simulink model "TST_Rail_MonMeUn"  (R2016b)
settings: Solver=FixedStepDiscrete  StartTime=0.0  StopTime=simTime  FixedStep=sampleTime  RelTol=1e-3
values from neighbouring files (symbols this model uses):
  testCase = 1    [initTST_Rail_MonMeUn_001.m]    (also in initTST_Rail_MonMeUn_002.m = 2; initTST_Rail_MonMeUn_003.m = 3; initTST_Rail_MonMeUn_004.m = 4; initTST_Rail_MonMeUn_005.m = 5)
libraries: simulink x91, UnitTest_Lib x81
(part 3 of 5)

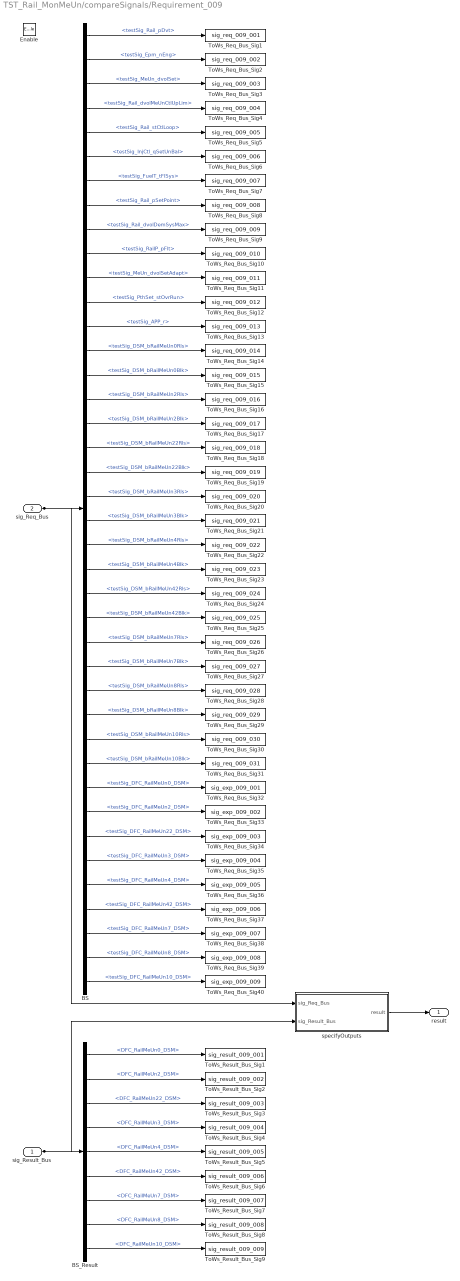
== system TST_Rail_MonMeUn/compareSignals/Requirement_009 ==
  sig_Result_Bus : Inport
  sig_Req_Bus : Inport  Port=2
  Enable : EnablePort
  BS : BusSelector  OutputSignals=testSig_Rail_pDvt,testSig_Epm_nEng,testSig_MeUn_dvolSet,testSig_Rail_dvolMeUnCtlUpLim,testSig_Rail_stCtlLoop,testSig_InjCtl_qSetUnBal,testSig_FuelT_tFlSys,testSig_Rail_pSetPoint,testSig_Rail_dvolDemSysMax,testSig_RailP_pFlt,testSig_MeUn_dvolSetAdapt,testSig_PthSet_stOvrRun,testSig_APP_r,testSig_DSM_bRailMeUn0Rls,testSig_DSM_bRailMeUn0Blk,testSig_DSM_bRailMeUn2Rls,testSig_DSM_bRailMeUn2Blk,testSig_DSM_bRailMeUn22Rls,testSig_DSM_bRailMeUn22Blk,testSig_DSM_bRailMeUn3Rls,testSig_DSM_bRailMeUn3Blk,testSig_DSM_bRailMeUn4Rls,testSig_DSM_bRailMeUn4Blk,testSig_DSM_bRailMeUn42Rls,testSig_DSM_bRailMeUn42Blk,testSig_DSM_bRailMeUn7Rls,testSig_DSM_bRailMeUn7Blk,testSig_DSM_bRailMeUn8Rls,testSig_DSM_bRailMeUn8Blk,testSig_DSM_bRailMeUn10Rls,testSig_DSM_bRailMeUn10Blk,testSig_DFC_RailMeUn0_DSM,testSig_DFC_RailMeUn2_DSM,testSig_DFC_RailMeUn22_DSM,testSig_DFC_RailMeUn3_DSM,testSig_DFC_RailMeUn4_DSM,testSig_DFC_RailMeUn42_DSM,testSig_DFC_RailMeUn7_DSM,testSig_DFC_RailMeUn8_DSM,testSig_DFC_RailMeUn10_DSM
  BS_Result : BusSelector  OutputSignals=DFC_RailMeUn0_DSM,DFC_RailMeUn2_DSM,DFC_RailMeUn22_DSM,DFC_RailMeUn3_DSM,DFC_RailMeUn4_DSM,DFC_RailMeUn42_DSM,DFC_RailMeUn7_DSM,DFC_RailMeUn8_DSM,DFC_RailMeUn10_DSM
  ToWs_Req_Bus_Sig1 : ToWorkspace  VariableName=sig_req_009_001  SaveFormat=Structure With Time
  ToWs_Req_Bus_Sig10 : ToWorkspace  VariableName=sig_req_009_010  SaveFormat=Structure With Time
  ToWs_Req_Bus_Sig11 : ToWorkspace  VariableName=sig_req_009_011  SaveFormat=Structure With Time
  ToWs_Req_Bus_Sig12 : ToWorkspace  VariableName=sig_req_009_012  SaveFormat=Structure With Time
  ToWs_Req_Bus_Sig13 : ToWorkspace  VariableName=sig_req_009_013  SaveFormat=Structure With Time
  ToWs_Req_Bus_Sig14 : ToWorkspace  VariableName=sig_req_009_014  SaveFormat=Structure With Time
  ToWs_Req_Bus_Sig15 : ToWorkspace  VariableName=sig_req_009_015  SaveFormat=Structure With Time
  ToWs_Req_Bus_Sig16 : ToWorkspace  VariableName=sig_req_009_016  SaveFormat=Structure With Time
  ToWs_Req_Bus_Sig17 : ToWorkspace  VariableName=sig_req_009_017  SaveFormat=Structure With Time
  ToWs_Req_Bus_Sig18 : ToWorkspace  VariableName=sig_req_009_018  SaveFormat=Structure With Time
  ToWs_Req_Bus_Sig19 : ToWorkspace  VariableName=sig_req_009_019  SaveFormat=Structure With Time
  ToWs_Req_Bus_Sig2 : ToWorkspace  VariableName=sig_req_009_002  SaveFormat=Structure With Time
  ToWs_Req_Bus_Sig20 : ToWorkspace  VariableName=sig_req_009_020  SaveFormat=Structure With Time
  ToWs_Req_Bus_Sig21 : ToWorkspace  VariableName=sig_req_009_021  SaveFormat=Structure With Time
  ToWs_Req_Bus_Sig22 : ToWorkspace  VariableName=sig_req_009_022  SaveFormat=Structure With Time
  ToWs_Req_Bus_Sig23 : ToWorkspace  VariableName=sig_req_009_023  SaveFormat=Structure With Time
  ToWs_Req_Bus_Sig24 : ToWorkspace  VariableName=sig_req_009_024  SaveFormat=Structure With Time
  ToWs_Req_Bus_Sig25 : ToWorkspace  VariableName=sig_req_009_025  SaveFormat=Structure With Time
  ToWs_Req_Bus_Sig26 : ToWorkspace  VariableName=sig_req_009_026  SaveFormat=Structure With Time
  ToWs_Req_Bus_Sig27 : ToWorkspace  VariableName=sig_req_009_027  SaveFormat=Structure With Time
  ToWs_Req_Bus_Sig28 : ToWorkspace  VariableName=sig_req_009_028  SaveFormat=Structure With Time
  ToWs_Req_Bus_Sig29 : ToWorkspace  VariableName=sig_req_009_029  SaveFormat=Structure With Time
  ToWs_Req_Bus_Sig3 : ToWorkspace  VariableName=sig_req_009_003  SaveFormat=Structure With Time
  ToWs_Req_Bus_Sig30 : ToWorkspace  VariableName=sig_req_009_030  SaveFormat=Structure With Time
  ToWs_Req_Bus_Sig31 : ToWorkspace  VariableName=sig_req_009_031  SaveFormat=Structure With Time
  ToWs_Req_Bus_Sig32 : ToWorkspace  VariableName=sig_exp_009_001  SaveFormat=Structure With Time
  ToWs_Req_Bus_Sig33 : ToWorkspace  VariableName=sig_exp_009_002  SaveFormat=Structure With Time
  ToWs_Req_Bus_Sig34 : ToWorkspace  VariableName=sig_exp_009_003  SaveFormat=Structure With Time
  ToWs_Req_Bus_Sig35 : ToWorkspace  VariableName=sig_exp_009_004  SaveFormat=Structure With Time
  ToWs_Req_Bus_Sig36 : ToWorkspace  VariableName=sig_exp_009_005  SaveFormat=Structure With Time
  ToWs_Req_Bus_Sig37 : ToWorkspace  VariableName=sig_exp_009_006  SaveFormat=Structure With Time
  ToWs_Req_Bus_Sig38 : ToWorkspace  VariableName=sig_exp_009_007  SaveFormat=Structure With Time
  ToWs_Req_Bus_Sig39 : ToWorkspace  VariableName=sig_exp_009_008  SaveFormat=Structure With Time
  ToWs_Req_Bus_Sig4 : ToWorkspace  VariableName=sig_req_009_004  SaveFormat=Structure With Time
  ToWs_Req_Bus_Sig40 : ToWorkspace  VariableName=sig_exp_009_009  SaveFormat=Structure With Time
  ToWs_Req_Bus_Sig5 : ToWorkspace  VariableName=sig_req_009_005  SaveFormat=Structure With Time
  ToWs_Req_Bus_Sig6 : ToWorkspace  VariableName=sig_req_009_006  SaveFormat=Structure With Time
  ToWs_Req_Bus_Sig7 : ToWorkspace  VariableName=sig_req_009_007  SaveFormat=Structure With Time
  ToWs_Req_Bus_Sig8 : ToWorkspace  VariableName=sig_req_009_008  SaveFormat=Structure With Time
  ToWs_Req_Bus_Sig9 : ToWorkspace  VariableName=sig_req_009_009  SaveFormat=Structure With Time
  ToWs_Result_Bus_Sig1 : ToWorkspace  VariableName=sig_result_009_001  SaveFormat=Structure With Time
  ToWs_Result_Bus_Sig2 : ToWorkspace  VariableName=sig_result_009_002  SaveFormat=Structure With Time
  ToWs_Result_Bus_Sig3 : ToWorkspace  VariableName=sig_result_009_003  SaveFormat=Structure With Time
  ToWs_Result_Bus_Sig4 : ToWorkspace  VariableName=sig_result_009_004  SaveFormat=Structure With Time
  ToWs_Result_Bus_Sig5 : ToWorkspace  VariableName=sig_result_009_005  SaveFormat=Structure With Time
  ToWs_Result_Bus_Sig6 : ToWorkspace  VariableName=sig_result_009_006  SaveFormat=Structure With Time
  ToWs_Result_Bus_Sig7 : ToWorkspace  VariableName=sig_result_009_007  SaveFormat=Structure With Time
  ToWs_Result_Bus_Sig8 : ToWorkspace  VariableName=sig_result_009_008  SaveFormat=Structure With Time
  ToWs_Result_Bus_Sig9 : ToWorkspace  VariableName=sig_result_009_009  SaveFormat=Structure With Time
  specifyOutputs : Subsystem
  result : Outport
  wires:
  sig_Req_Bus/1 -> BS/1, specifyOutputs/1(sig_Req_Bus)
  BS/1 -> ToWs_Req_Bus_Sig1/1  "<testSig_Rail_pDvt>"
  BS/2 -> ToWs_Req_Bus_Sig2/1  "<testSig_Epm_nEng>"
  BS/3 -> ToWs_Req_Bus_Sig3/1  "<testSig_MeUn_dvolSet>"
  BS/4 -> ToWs_Req_Bus_Sig4/1  "<testSig_Rail_dvolMeUnCtlUpLim>"
  BS/5 -> ToWs_Req_Bus_Sig5/1  "<testSig_Rail_stCtlLoop>"
  BS/6 -> ToWs_Req_Bus_Sig6/1  "<testSig_InjCtl_qSetUnBal>"
  BS/7 -> ToWs_Req_Bus_Sig7/1  "<testSig_FuelT_tFlSys>"
  BS/8 -> ToWs_Req_Bus_Sig8/1  "<testSig_Rail_pSetPoint>"
  BS/9 -> ToWs_Req_Bus_Sig9/1  "<testSig_Rail_dvolDemSysMax>"
  BS/10 -> ToWs_Req_Bus_Sig10/1  "<testSig_RailP_pFlt>"
  BS/11 -> ToWs_Req_Bus_Sig11/1  "<testSig_MeUn_dvolSetAdapt>"
  BS/12 -> ToWs_Req_Bus_Sig12/1  "<testSig_PthSet_stOvrRun>"
  BS/13 -> ToWs_Req_Bus_Sig13/1  "<testSig_APP_r>"
  BS/14 -> ToWs_Req_Bus_Sig14/1  "<testSig_DSM_bRailMeUn0Rls>"
  BS/15 -> ToWs_Req_Bus_Sig15/1  "<testSig_DSM_bRailMeUn0Blk>"
  BS/16 -> ToWs_Req_Bus_Sig16/1  "<testSig_DSM_bRailMeUn2Rls>"
  BS/17 -> ToWs_Req_Bus_Sig17/1  "<testSig_DSM_bRailMeUn2Blk>"
  BS/18 -> ToWs_Req_Bus_Sig18/1  "<testSig_DSM_bRailMeUn22Rls>"
  BS/19 -> ToWs_Req_Bus_Sig19/1  "<testSig_DSM_bRailMeUn22Blk>"
  BS/20 -> ToWs_Req_Bus_Sig20/1  "<testSig_DSM_bRailMeUn3Rls>"
  BS/21 -> ToWs_Req_Bus_Sig21/1  "<testSig_DSM_bRailMeUn3Blk>"
  BS/22 -> ToWs_Req_Bus_Sig22/1  "<testSig_DSM_bRailMeUn4Rls>"
  BS/23 -> ToWs_Req_Bus_Sig23/1  "<testSig_DSM_bRailMeUn4Blk>"
  BS/24 -> ToWs_Req_Bus_Sig24/1  "<testSig_DSM_bRailMeUn42Rls>"
  BS/25 -> ToWs_Req_Bus_Sig25/1  "<testSig_DSM_bRailMeUn42Blk>"
  BS/26 -> ToWs_Req_Bus_Sig26/1  "<testSig_DSM_bRailMeUn7Rls>"
  BS/27 -> ToWs_Req_Bus_Sig27/1  "<testSig_DSM_bRailMeUn7Blk>"
  BS/28 -> ToWs_Req_Bus_Sig28/1  "<testSig_DSM_bRailMeUn8Rls>"
  BS/29 -> ToWs_Req_Bus_Sig29/1  "<testSig_DSM_bRailMeUn8Blk>"
  BS/30 -> ToWs_Req_Bus_Sig30/1  "<testSig_DSM_bRailMeUn10Rls>"
  BS/31 -> ToWs_Req_Bus_Sig31/1  "<testSig_DSM_bRailMeUn10Blk>"
  BS/32 -> ToWs_Req_Bus_Sig32/1  "<testSig_DFC_RailMeUn0_DSM>"
  BS/33 -> ToWs_Req_Bus_Sig33/1  "<testSig_DFC_RailMeUn2_DSM>"
  BS/34 -> ToWs_Req_Bus_Sig34/1  "<testSig_DFC_RailMeUn22_DSM>"
  BS/35 -> ToWs_Req_Bus_Sig35/1  "<testSig_DFC_RailMeUn3_DSM>"
  BS/36 -> ToWs_Req_Bus_Sig36/1  "<testSig_DFC_RailMeUn4_DSM>"
  BS/37 -> ToWs_Req_Bus_Sig37/1  "<testSig_DFC_RailMeUn42_DSM>"
  BS/38 -> ToWs_Req_Bus_Sig38/1  "<testSig_DFC_RailMeUn7_DSM>"
  BS/39 -> ToWs_Req_Bus_Sig39/1  "<testSig_DFC_RailMeUn8_DSM>"
  BS/40 -> ToWs_Req_Bus_Sig40/1  "<testSig_DFC_RailMeUn10_DSM>"
  sig_Result_Bus/1 -> BS_Result/1, specifyOutputs/2(sig_Result_Bus)
  BS_Result/1 -> ToWs_Result_Bus_Sig1/1  "<DFC_RailMeUn0_DSM>"
  BS_Result/2 -> ToWs_Result_Bus_Sig2/1  "<DFC_RailMeUn2_DSM>"
  BS_Result/3 -> ToWs_Result_Bus_Sig3/1  "<DFC_RailMeUn22_DSM>"
  BS_Result/4 -> ToWs_Result_Bus_Sig4/1  "<DFC_RailMeUn3_DSM>"
  BS_Result/5 -> ToWs_Result_Bus_Sig5/1  "<DFC_RailMeUn4_DSM>"
  BS_Result/6 -> ToWs_Result_Bus_Sig6/1  "<DFC_RailMeUn42_DSM>"
  BS_Result/7 -> ToWs_Result_Bus_Sig7/1  "<DFC_RailMeUn7_DSM>"
  BS_Result/8 -> ToWs_Result_Bus_Sig8/1  "<DFC_RailMeUn8_DSM>"
  BS_Result/9 -> ToWs_Result_Bus_Sig9/1  "<DFC_RailMeUn10_DSM>"
  specifyOutputs/1(result) -> result/1

== system TST_Rail_MonMeUn/simulationInput/testSignals_R001 ==
  BC : BusCreator  Inputs=40
  spec_APP_r : FromWorkspace  VariableName=testSig_APP_r  Interpolate=off  OutputAfterFinalValue=Holding final value
  spec_DFC_RailMeUn0_DSM : FromWorkspace  VariableName=testSig_DFC_RailMeUn0_DSM  Interpolate=off  OutputAfterFinalValue=Holding final value
  spec_DFC_RailMeUn10_DSM : FromWorkspace  VariableName=testSig_DFC_RailMeUn10_DSM  Interpolate=off  OutputAfterFinalValue=Holding final value
  spec_DFC_RailMeUn22_DSM : FromWorkspace  VariableName=testSig_DFC_RailMeUn22_DSM  Interpolate=off  OutputAfterFinalValue=Holding final value
  spec_DFC_RailMeUn2_DSM : FromWorkspace  VariableName=testSig_DFC_RailMeUn2_DSM  Interpolate=off  OutputAfterFinalValue=Holding final value
  spec_DFC_RailMeUn3_DSM : FromWorkspace  VariableName=testSig_DFC_RailMeUn3_DSM  Interpolate=off  OutputAfterFinalValue=Holding final value
  spec_DFC_RailMeUn42_DSM : FromWorkspace  VariableName=testSig_DFC_RailMeUn42_DSM  Interpolate=off  OutputAfterFinalValue=Holding final value
  spec_DFC_RailMeUn4_DSM : FromWorkspace  VariableName=testSig_DFC_RailMeUn4_DSM  Interpolate=off  OutputAfterFinalValue=Holding final value
  spec_DFC_RailMeUn7_DSM : FromWorkspace  VariableName=testSig_DFC_RailMeUn7_DSM  Interpolate=off  OutputAfterFinalValue=Holding final value
  spec_DFC_RailMeUn8_DSM : FromWorkspace  VariableName=testSig_DFC_RailMeUn8_DSM  Interpolate=off  OutputAfterFinalValue=Holding final value
  spec_DSM_bRailMeUn0Blk : FromWorkspace  VariableName=testSig_DSM_bRailMeUn0Blk  Interpolate=off  OutputAfterFinalValue=Holding final value
  spec_DSM_bRailMeUn0Rls : FromWorkspace  VariableName=testSig_DSM_bRailMeUn0Rls  Interpolate=off  OutputAfterFinalValue=Holding final value
  spec_DSM_bRailMeUn10Blk : FromWorkspace  VariableName=testSig_DSM_bRailMeUn10Blk  Interpolate=off  OutputAfterFinalValue=Holding final value
  spec_DSM_bRailMeUn10Rls : FromWorkspace  VariableName=testSig_DSM_bRailMeUn10Rls  Interpolate=off  OutputAfterFinalValue=Holding final value
  spec_DSM_bRailMeUn22Blk : FromWorkspace  VariableName=testSig_DSM_bRailMeUn22Blk  Interpolate=off  OutputAfterFinalValue=Holding final value
  spec_DSM_bRailMeUn22Rls : FromWorkspace  VariableName=testSig_DSM_bRailMeUn22Rls  Interpolate=off  OutputAfterFinalValue=Holding final value
  spec_DSM_bRailMeUn2Blk : FromWorkspace  VariableName=testSig_DSM_bRailMeUn2Blk  Interpolate=off  OutputAfterFinalValue=Holding final value
  spec_DSM_bRailMeUn2Rls : FromWorkspace  VariableName=testSig_DSM_bRailMeUn2Rls  Interpolate=off  OutputAfterFinalValue=Holding final value
  spec_DSM_bRailMeUn3Blk : FromWorkspace  VariableName=testSig_DSM_bRailMeUn3Blk  Interpolate=off  OutputAfterFinalValue=Holding final value
  spec_DSM_bRailMeUn3Rls : FromWorkspace  VariableName=testSig_DSM_bRailMeUn3Rls  Interpolate=off  OutputAfterFinalValue=Holding final value
  spec_DSM_bRailMeUn42Blk : FromWorkspace  VariableName=testSig_DSM_bRailMeUn42Blk  Interpolate=off  OutputAfterFinalValue=Holding final value
  spec_DSM_bRailMeUn42Rls : FromWorkspace  VariableName=testSig_DSM_bRailMeUn42Rls  Interpolate=off  OutputAfterFinalValue=Holding final value
  spec_DSM_bRailMeUn4Blk : FromWorkspace  VariableName=testSig_DSM_bRailMeUn4Blk  Interpolate=off  OutputAfterFinalValue=Holding final value
  spec_DSM_bRailMeUn4Rls : FromWorkspace  VariableName=testSig_DSM_bRailMeUn4Rls  Interpolate=off  OutputAfterFinalValue=Holding final value
  spec_DSM_bRailMeUn7Blk : FromWorkspace  VariableName=testSig_DSM_bRailMeUn7Blk  Interpolate=off  OutputAfterFinalValue=Holding final value
  spec_DSM_bRailMeUn7Rls : FromWorkspace  VariableName=testSig_DSM_bRailMeUn7Rls  Interpolate=off  OutputAfterFinalValue=Holding final value
  spec_DSM_bRailMeUn8Blk : FromWorkspace  VariableName=testSig_DSM_bRailMeUn8Blk  Interpolate=off  OutputAfterFinalValue=Holding final value
  spec_DSM_bRailMeUn8Rls : FromWorkspace  VariableName=testSig_DSM_bRailMeUn8Rls  Interpolate=off  OutputAfterFinalValue=Holding final value
  spec_Epm_nEng : FromWorkspace  VariableName=testSig_Epm_nEng  Interpolate=off  OutputAfterFinalValue=Holding final value
  spec_FuelT_tFlSys : FromWorkspace  VariableName=testSig_FuelT_tFlSys  Interpolate=off  OutputAfterFinalValue=Holding final value
  spec_InjCtl_qSetUnBal : FromWorkspace  VariableName=testSig_InjCtl_qSetUnBal  Interpolate=off  OutputAfterFinalValue=Holding final value
  spec_MeUn_dvolSet : FromWorkspace  VariableName=testSig_MeUn_dvolSet  Interpolate=off  OutputAfterFinalValue=Holding final value
  spec_MeUn_dvolSetAdapt : FromWorkspace  VariableName=testSig_MeUn_dvolSetAdapt  Interpolate=off  OutputAfterFinalValue=Holding final value
  spec_PthSet_stOvrRun : FromWorkspace  VariableName=testSig_PthSet_stOvrRun  Interpolate=off  OutputAfterFinalValue=Holding final value
  spec_RailP_pFlt : FromWorkspace  VariableName=testSig_RailP_pFlt  Interpolate=off  OutputAfterFinalValue=Holding final value
  spec_Rail_dvolDemSysMax : FromWorkspace  VariableName=testSig_Rail_dvolDemSysMax  Interpolate=off  OutputAfterFinalValue=Holding final value
  spec_Rail_dvolMeUnCtlUpLim : FromWorkspace  VariableName=testSig_Rail_dvolMeUnCtlUpLim  Interpolate=off  OutputAfterFinalValue=Holding final value
  spec_Rail_pDvt : FromWorkspace  VariableName=testSig_Rail_pDvt  Interpolate=off  OutputAfterFinalValue=Holding final value
  spec_Rail_pSetPoint : FromWorkspace  VariableName=testSig_Rail_pSetPoint  Interpolate=off  OutputAfterFinalValue=Holding final value
  spec_Rail_stCtlLoop : FromWorkspace  VariableName=testSig_Rail_stCtlLoop  Interpolate=off  OutputAfterFinalValue=Holding final value
  testSignals : Outport
  wires:
  BC/1 -> testSignals/1
  spec_Rail_pDvt/1 -> BC/1  "testSig_Rail_pDvt"
  spec_Epm_nEng/1 -> BC/2  "testSig_Epm_nEng"
  spec_MeUn_dvolSet/1 -> BC/3  "testSig_MeUn_dvolSet"
  spec_Rail_dvolMeUnCtlUpLim/1 -> BC/4  "testSig_Rail_dvolMeUnCtlUpLim"
  spec_Rail_stCtlLoop/1 -> BC/5  "testSig_Rail_stCtlLoop"
  spec_InjCtl_qSetUnBal/1 -> BC/6  "testSig_InjCtl_qSetUnBal"
  spec_FuelT_tFlSys/1 -> BC/7  "testSig_FuelT_tFlSys"
  spec_Rail_pSetPoint/1 -> BC/8  "testSig_Rail_pSetPoint"
  spec_Rail_dvolDemSysMax/1 -> BC/9  "testSig_Rail_dvolDemSysMax"
  spec_RailP_pFlt/1 -> BC/10  "testSig_RailP_pFlt"
  spec_MeUn_dvolSetAdapt/1 -> BC/11  "testSig_MeUn_dvolSetAdapt"
  spec_PthSet_stOvrRun/1 -> BC/12  "testSig_PthSet_stOvrRun"
  spec_APP_r/1 -> BC/13  "testSig_APP_r"
  spec_DSM_bRailMeUn0Rls/1 -> BC/14  "testSig_DSM_bRailMeUn0Rls"
  spec_DSM_bRailMeUn0Blk/1 -> BC/15  "testSig_DSM_bRailMeUn0Blk"
  spec_DSM_bRailMeUn2Rls/1 -> BC/16  "testSig_DSM_bRailMeUn2Rls"
  spec_DSM_bRailMeUn2Blk/1 -> BC/17  "testSig_DSM_bRailMeUn2Blk"
  spec_DSM_bRailMeUn22Rls/1 -> BC/18  "testSig_DSM_bRailMeUn22Rls"
  spec_DSM_bRailMeUn22Blk/1 -> BC/19  "testSig_DSM_bRailMeUn22Blk"
  spec_DSM_bRailMeUn3Rls/1 -> BC/20  "testSig_DSM_bRailMeUn3Rls"
  spec_DSM_bRailMeUn3Blk/1 -> BC/21  "testSig_DSM_bRailMeUn3Blk"
  spec_DSM_bRailMeUn4Rls/1 -> BC/22  "testSig_DSM_bRailMeUn4Rls"
  spec_DSM_bRailMeUn4Blk/1 -> BC/23  "testSig_DSM_bRailMeUn4Blk"
  spec_DSM_bRailMeUn42Rls/1 -> BC/24  "testSig_DSM_bRailMeUn42Rls"
  spec_DSM_bRailMeUn42Blk/1 -> BC/25  "testSig_DSM_bRailMeUn42Blk"
  spec_DSM_bRailMeUn7Rls/1 -> BC/26  "testSig_DSM_bRailMeUn7Rls"
  spec_DSM_bRailMeUn7Blk/1 -> BC/27  "testSig_DSM_bRailMeUn7Blk"
  spec_DSM_bRailMeUn8Rls/1 -> BC/28  "testSig_DSM_bRailMeUn8Rls"
  spec_DSM_bRailMeUn8Blk/1 -> BC/29  "testSig_DSM_bRailMeUn8Blk"
  spec_DSM_bRailMeUn10Rls/1 -> BC/30  "testSig_DSM_bRailMeUn10Rls"
  spec_DSM_bRailMeUn10Blk/1 -> BC/31  "testSig_DSM_bRailMeUn10Blk"
  spec_DFC_RailMeUn0_DSM/1 -> BC/32  "testSig_DFC_RailMeUn0_DSM"
  spec_DFC_RailMeUn2_DSM/1 -> BC/33  "testSig_DFC_RailMeUn2_DSM"
  spec_DFC_RailMeUn22_DSM/1 -> BC/34  "testSig_DFC_RailMeUn22_DSM"
  spec_DFC_RailMeUn3_DSM/1 -> BC/35  "testSig_DFC_RailMeUn3_DSM"
  spec_DFC_RailMeUn4_DSM/1 -> BC/36  "testSig_DFC_RailMeUn4_DSM"
  spec_DFC_RailMeUn42_DSM/1 -> BC/37  "testSig_DFC_RailMeUn42_DSM"
  spec_DFC_RailMeUn7_DSM/1 -> BC/38  "testSig_DFC_RailMeUn7_DSM"
  spec_DFC_RailMeUn8_DSM/1 -> BC/39  "testSig_DFC_RailMeUn8_DSM"
  spec_DFC_RailMeUn10_DSM/1 -> BC/40  "testSig_DFC_RailMeUn10_DSM"

== system TST_Rail_MonMeUn/simulationInput/testSignals_R002 ==
  BC : BusCreator  Inputs=40
  spec_APP_r : FromWorkspace  VariableName=testSig_APP_r  Interpolate=off  OutputAfterFinalValue=Holding final value
  spec_DFC_RailMeUn0_DSM : FromWorkspace  VariableName=testSig_DFC_RailMeUn0_DSM  Interpolate=off  OutputAfterFinalValue=Holding final value
  spec_DFC_RailMeUn10_DSM : FromWorkspace  VariableName=testSig_DFC_RailMeUn10_DSM  Interpolate=off  OutputAfterFinalValue=Holding final value
  spec_DFC_RailMeUn22_DSM : FromWorkspace  VariableName=testSig_DFC_RailMeUn22_DSM  Interpolate=off  OutputAfterFinalValue=Holding final value
  spec_DFC_RailMeUn2_DSM : FromWorkspace  VariableName=testSig_DFC_RailMeUn2_DSM  Interpolate=off  OutputAfterFinalValue=Holding final value
  spec_DFC_RailMeUn3_DSM : FromWorkspace  VariableName=testSig_DFC_RailMeUn3_DSM  Interpolate=off  OutputAfterFinalValue=Holding final value
  spec_DFC_RailMeUn42_DSM : FromWorkspace  VariableName=testSig_DFC_RailMeUn42_DSM  Interpolate=off  OutputAfterFinalValue=Holding final value
  spec_DFC_RailMeUn4_DSM : FromWorkspace  VariableName=testSig_DFC_RailMeUn4_DSM  Interpolate=off  OutputAfterFinalValue=Holding final value
  spec_DFC_RailMeUn7_DSM : FromWorkspace  VariableName=testSig_DFC_RailMeUn7_DSM  Interpolate=off  OutputAfterFinalValue=Holding final value
  spec_DFC_RailMeUn8_DSM : FromWorkspace  VariableName=testSig_DFC_RailMeUn8_DSM  Interpolate=off  OutputAfterFinalValue=Holding final value
  spec_DSM_bRailMeUn0Blk : FromWorkspace  VariableName=testSig_DSM_bRailMeUn0Blk  Interpolate=off  OutputAfterFinalValue=Holding final value
  spec_DSM_bRailMeUn0Rls : FromWorkspace  VariableName=testSig_DSM_bRailMeUn0Rls  Interpolate=off  OutputAfterFinalValue=Holding final value
  spec_DSM_bRailMeUn10Blk : FromWorkspace  VariableName=testSig_DSM_bRailMeUn10Blk  Interpolate=off  OutputAfterFinalValue=Holding final value
  spec_DSM_bRailMeUn10Rls : FromWorkspace  VariableName=testSig_DSM_bRailMeUn10Rls  Interpolate=off  OutputAfterFinalValue=Holding final value
  spec_DSM_bRailMeUn22Blk : FromWorkspace  VariableName=testSig_DSM_bRailMeUn22Blk  Interpolate=off  OutputAfterFinalValue=Holding final value
  spec_DSM_bRailMeUn22Rls : FromWorkspace  VariableName=testSig_DSM_bRailMeUn22Rls  Interpolate=off  OutputAfterFinalValue=Holding final value
  spec_DSM_bRailMeUn2Blk : FromWorkspace  VariableName=testSig_DSM_bRailMeUn2Blk  Interpolate=off  OutputAfterFinalValue=Holding final value
  spec_DSM_bRailMeUn2Rls : FromWorkspace  VariableName=testSig_DSM_bRailMeUn2Rls  Interpolate=off  OutputAfterFinalValue=Holding final value
  spec_DSM_bRailMeUn3Blk : FromWorkspace  VariableName=testSig_DSM_bRailMeUn3Blk  Interpolate=off  OutputAfterFinalValue=Holding final value
  spec_DSM_bRailMeUn3Rls : FromWorkspace  VariableName=testSig_DSM_bRailMeUn3Rls  Interpolate=off  OutputAfterFinalValue=Holding final value
  spec_DSM_bRailMeUn42Blk : FromWorkspace  VariableName=testSig_DSM_bRailMeUn42Blk  Interpolate=off  OutputAfterFinalValue=Holding final value
  spec_DSM_bRailMeUn42Rls : FromWorkspace  VariableName=testSig_DSM_bRailMeUn42Rls  Interpolate=off  OutputAfterFinalValue=Holding final value
  spec_DSM_bRailMeUn4Blk : FromWorkspace  VariableName=testSig_DSM_bRailMeUn4Blk  Interpolate=off  OutputAfterFinalValue=Holding final value
  spec_DSM_bRailMeUn4Rls : FromWorkspace  VariableName=testSig_DSM_bRailMeUn4Rls  Interpolate=off  OutputAfterFinalValue=Holding final value
  spec_DSM_bRailMeUn7Blk : FromWorkspace  VariableName=testSig_DSM_bRailMeUn7Blk  Interpolate=off  OutputAfterFinalValue=Holding final value
  spec_DSM_bRailMeUn7Rls : FromWorkspace  VariableName=testSig_DSM_bRailMeUn7Rls  Interpolate=off  OutputAfterFinalValue=Holding final value
  spec_DSM_bRailMeUn8Blk : FromWorkspace  VariableName=testSig_DSM_bRailMeUn8Blk  Interpolate=off  OutputAfterFinalValue=Holding final value
  spec_DSM_bRailMeUn8Rls : FromWorkspace  VariableName=testSig_DSM_bRailMeUn8Rls  Interpolate=off  OutputAfterFinalValue=Holding final value
  spec_Epm_nEng : FromWorkspace  VariableName=testSig_Epm_nEng  Interpolate=off  OutputAfterFinalValue=Holding final value
  spec_FuelT_tFlSys : FromWorkspace  VariableName=testSig_FuelT_tFlSys  Interpolate=off  OutputAfterFinalValue=Holding final value
  spec_InjCtl_qSetUnBal : FromWorkspace  VariableName=testSig_InjCtl_qSetUnBal  Interpolate=off  OutputAfterFinalValue=Holding final value
  spec_MeUn_dvolSet : FromWorkspace  VariableName=testSig_MeUn_dvolSet  Interpolate=off  OutputAfterFinalValue=Holding final value
  spec_MeUn_dvolSetAdapt : FromWorkspace  VariableName=testSig_MeUn_dvolSetAdapt  Interpolate=off  OutputAfterFinalValue=Holding final value
  spec_PthSet_stOvrRun : FromWorkspace  VariableName=testSig_PthSet_stOvrRun  Interpolate=off  OutputAfterFinalValue=Holding final value
  spec_RailP_pFlt : FromWorkspace  VariableName=testSig_RailP_pFlt  Interpolate=off  OutputAfterFinalValue=Holding final value
  spec_Rail_dvolDemSysMax : FromWorkspace  VariableName=testSig_Rail_dvolDemSysMax  Interpolate=off  OutputAfterFinalValue=Holding final value
  spec_Rail_dvolMeUnCtlUpLim : FromWorkspace  VariableName=testSig_Rail_dvolMeUnCtlUpLim  Interpolate=off  OutputAfterFinalValue=Holding final value
  spec_Rail_pDvt : FromWorkspace  VariableName=testSig_Rail_pDvt  Interpolate=off  OutputAfterFinalValue=Holding final value
  spec_Rail_pSetPoint : FromWorkspace  VariableName=testSig_Rail_pSetPoint  Interpolate=off  OutputAfterFinalValue=Holding final value
  spec_Rail_stCtlLoop : FromWorkspace  VariableName=testSig_Rail_stCtlLoop  Interpolate=off  OutputAfterFinalValue=Holding final value
  testSignals : Outport
  wires:
  BC/1 -> testSignals/1
  spec_Rail_pDvt/1 -> BC/1  "testSig_Rail_pDvt"
  spec_Epm_nEng/1 -> BC/2  "testSig_Epm_nEng"
  spec_MeUn_dvolSet/1 -> BC/3  "testSig_MeUn_dvolSet"
  spec_Rail_dvolMeUnCtlUpLim/1 -> BC/4  "testSig_Rail_dvolMeUnCtlUpLim"
  spec_Rail_stCtlLoop/1 -> BC/5  "testSig_Rail_stCtlLoop"
  spec_InjCtl_qSetUnBal/1 -> BC/6  "testSig_InjCtl_qSetUnBal"
  spec_FuelT_tFlSys/1 -> BC/7  "testSig_FuelT_tFlSys"
  spec_Rail_pSetPoint/1 -> BC/8  "testSig_Rail_pSetPoint"
  spec_Rail_dvolDemSysMax/1 -> BC/9  "testSig_Rail_dvolDemSysMax"
  spec_RailP_pFlt/1 -> BC/10  "testSig_RailP_pFlt"
  spec_MeUn_dvolSetAdapt/1 -> BC/11  "testSig_MeUn_dvolSetAdapt"
  spec_PthSet_stOvrRun/1 -> BC/12  "testSig_PthSet_stOvrRun"
  spec_APP_r/1 -> BC/13  "testSig_APP_r"
  spec_DSM_bRailMeUn0Rls/1 -> BC/14  "testSig_DSM_bRailMeUn0Rls"
  spec_DSM_bRailMeUn0Blk/1 -> BC/15  "testSig_DSM_bRailMeUn0Blk"
  spec_DSM_bRailMeUn2Rls/1 -> BC/16  "testSig_DSM_bRailMeUn2Rls"
  spec_DSM_bRailMeUn2Blk/1 -> BC/17  "testSig_DSM_bRailMeUn2Blk"
  spec_DSM_bRailMeUn22Rls/1 -> BC/18  "testSig_DSM_bRailMeUn22Rls"
  spec_DSM_bRailMeUn22Blk/1 -> BC/19  "testSig_DSM_bRailMeUn22Blk"
  spec_DSM_bRailMeUn3Rls/1 -> BC/20  "testSig_DSM_bRailMeUn3Rls"
  spec_DSM_bRailMeUn3Blk/1 -> BC/21  "testSig_DSM_bRailMeUn3Blk"
  spec_DSM_bRailMeUn4Rls/1 -> BC/22  "testSig_DSM_bRailMeUn4Rls"
  spec_DSM_bRailMeUn4Blk/1 -> BC/23  "testSig_DSM_bRailMeUn4Blk"
  spec_DSM_bRailMeUn42Rls/1 -> BC/24  "testSig_DSM_bRailMeUn42Rls"
  spec_DSM_bRailMeUn42Blk/1 -> BC/25  "testSig_DSM_bRailMeUn42Blk"
  spec_DSM_bRailMeUn7Rls/1 -> BC/26  "testSig_DSM_bRailMeUn7Rls"
  spec_DSM_bRailMeUn7Blk/1 -> BC/27  "testSig_DSM_bRailMeUn7Blk"
  spec_DSM_bRailMeUn8Rls/1 -> BC/28  "testSig_DSM_bRailMeUn8Rls"
  spec_DSM_bRailMeUn8Blk/1 -> BC/29  "testSig_DSM_bRailMeUn8Blk"
  spec_DSM_bRailMeUn10Rls/1 -> BC/30  "testSig_DSM_bRailMeUn10Rls"
  spec_DSM_bRailMeUn10Blk/1 -> BC/31  "testSig_DSM_bRailMeUn10Blk"
  spec_DFC_RailMeUn0_DSM/1 -> BC/32  "testSig_DFC_RailMeUn0_DSM"
  spec_DFC_RailMeUn2_DSM/1 -> BC/33  "testSig_DFC_RailMeUn2_DSM"
  spec_DFC_RailMeUn22_DSM/1 -> BC/34  "testSig_DFC_RailMeUn22_DSM"
  spec_DFC_RailMeUn3_DSM/1 -> BC/35  "testSig_DFC_RailMeUn3_DSM"
  spec_DFC_RailMeUn4_DSM/1 -> BC/36  "testSig_DFC_RailMeUn4_DSM"
  spec_DFC_RailMeUn42_DSM/1 -> BC/37  "testSig_DFC_RailMeUn42_DSM"
  spec_DFC_RailMeUn7_DSM/1 -> BC/38  "testSig_DFC_RailMeUn7_DSM"
  spec_DFC_RailMeUn8_DSM/1 -> BC/39  "testSig_DFC_RailMeUn8_DSM"
  spec_DFC_RailMeUn10_DSM/1 -> BC/40  "testSig_DFC_RailMeUn10_DSM"

== system TST_Rail_MonMeUn/simulationInput/testSignals_R003 ==
  BC : BusCreator  Inputs=40
  spec_APP_r : FromWorkspace  VariableName=testSig_APP_r  Interpolate=off  OutputAfterFinalValue=Holding final value
  spec_DFC_RailMeUn0_DSM : FromWorkspace  VariableName=testSig_DFC_RailMeUn0_DSM  Interpolate=off  OutputAfterFinalValue=Holding final value
  spec_DFC_RailMeUn10_DSM : FromWorkspace  VariableName=testSig_DFC_RailMeUn10_DSM  Interpolate=off  OutputAfterFinalValue=Holding final value
  spec_DFC_RailMeUn22_DSM : FromWorkspace  VariableName=testSig_DFC_RailMeUn22_DSM  Interpolate=off  OutputAfterFinalValue=Holding final value
  spec_DFC_RailMeUn2_DSM : FromWorkspace  VariableName=testSig_DFC_RailMeUn2_DSM  Interpolate=off  OutputAfterFinalValue=Holding final value
  spec_DFC_RailMeUn3_DSM : FromWorkspace  VariableName=testSig_DFC_RailMeUn3_DSM  Interpolate=off  OutputAfterFinalValue=Holding final value
  spec_DFC_RailMeUn42_DSM : FromWorkspace  VariableName=testSig_DFC_RailMeUn42_DSM  Interpolate=off  OutputAfterFinalValue=Holding final value
  spec_DFC_RailMeUn4_DSM : FromWorkspace  VariableName=testSig_DFC_RailMeUn4_DSM  Interpolate=off  OutputAfterFinalValue=Holding final value
  spec_DFC_RailMeUn7_DSM : FromWorkspace  VariableName=testSig_DFC_RailMeUn7_DSM  Interpolate=off  OutputAfterFinalValue=Holding final value
  spec_DFC_RailMeUn8_DSM : FromWorkspace  VariableName=testSig_DFC_RailMeUn8_DSM  Interpolate=off  OutputAfterFinalValue=Holding final value
  spec_DSM_bRailMeUn0Blk : FromWorkspace  VariableName=testSig_DSM_bRailMeUn0Blk  Interpolate=off  OutputAfterFinalValue=Holding final value
  spec_DSM_bRailMeUn0Rls : FromWorkspace  VariableName=testSig_DSM_bRailMeUn0Rls  Interpolate=off  OutputAfterFinalValue=Holding final value
  spec_DSM_bRailMeUn10Blk : FromWorkspace  VariableName=testSig_DSM_bRailMeUn10Blk  Interpolate=off  OutputAfterFinalValue=Holding final value
  spec_DSM_bRailMeUn10Rls : FromWorkspace  VariableName=testSig_DSM_bRailMeUn10Rls  Interpolate=off  OutputAfterFinalValue=Holding final value
  spec_DSM_bRailMeUn22Blk : FromWorkspace  VariableName=testSig_DSM_bRailMeUn22Blk  Interpolate=off  OutputAfterFinalValue=Holding final value
  spec_DSM_bRailMeUn22Rls : FromWorkspace  VariableName=testSig_DSM_bRailMeUn22Rls  Interpolate=off  OutputAfterFinalValue=Holding final value
  spec_DSM_bRailMeUn2Blk : FromWorkspace  VariableName=testSig_DSM_bRailMeUn2Blk  Interpolate=off  OutputAfterFinalValue=Holding final value
  spec_DSM_bRailMeUn2Rls : FromWorkspace  VariableName=testSig_DSM_bRailMeUn2Rls  Interpolate=off  OutputAfterFinalValue=Holding final value
  spec_DSM_bRailMeUn3Blk : FromWorkspace  VariableName=testSig_DSM_bRailMeUn3Blk  Interpolate=off  OutputAfterFinalValue=Holding final value
  spec_DSM_bRailMeUn3Rls : FromWorkspace  VariableName=testSig_DSM_bRailMeUn3Rls  Interpolate=off  OutputAfterFinalValue=Holding final value
  spec_DSM_bRailMeUn42Blk : FromWorkspace  VariableName=testSig_DSM_bRailMeUn42Blk  Interpolate=off  OutputAfterFinalValue=Holding final value
  spec_DSM_bRailMeUn42Rls : FromWorkspace  VariableName=testSig_DSM_bRailMeUn42Rls  Interpolate=off  OutputAfterFinalValue=Holding final value
  spec_DSM_bRailMeUn4Blk : FromWorkspace  VariableName=testSig_DSM_bRailMeUn4Blk  Interpolate=off  OutputAfterFinalValue=Holding final value
  spec_DSM_bRailMeUn4Rls : FromWorkspace  VariableName=testSig_DSM_bRailMeUn4Rls  Interpolate=off  OutputAfterFinalValue=Holding final value
  spec_DSM_bRailMeUn7Blk : FromWorkspace  VariableName=testSig_DSM_bRailMeUn7Blk  Interpolate=off  OutputAfterFinalValue=Holding final value
  spec_DSM_bRailMeUn7Rls : FromWorkspace  VariableName=testSig_DSM_bRailMeUn7Rls  Interpolate=off  OutputAfterFinalValue=Holding final value
  spec_DSM_bRailMeUn8Blk : FromWorkspace  VariableName=testSig_DSM_bRailMeUn8Blk  Interpolate=off  OutputAfterFinalValue=Holding final value
  spec_DSM_bRailMeUn8Rls : FromWorkspace  VariableName=testSig_DSM_bRailMeUn8Rls  Interpolate=off  OutputAfterFinalValue=Holding final value
  spec_Epm_nEng : FromWorkspace  VariableName=testSig_Epm_nEng  Interpolate=off  OutputAfterFinalValue=Holding final value
  spec_FuelT_tFlSys : FromWorkspace  VariableName=testSig_FuelT_tFlSys  Interpolate=off  OutputAfterFinalValue=Holding final value
  spec_InjCtl_qSetUnBal : FromWorkspace  VariableName=testSig_InjCtl_qSetUnBal  Interpolate=off  OutputAfterFinalValue=Holding final value
  spec_MeUn_dvolSet : FromWorkspace  VariableName=testSig_MeUn_dvolSet  Interpolate=off  OutputAfterFinalValue=Holding final value
  spec_MeUn_dvolSetAdapt : FromWorkspace  VariableName=testSig_MeUn_dvolSetAdapt  Interpolate=off  OutputAfterFinalValue=Holding final value
  spec_PthSet_stOvrRun : FromWorkspace  VariableName=testSig_PthSet_stOvrRun  Interpolate=off  OutputAfterFinalValue=Holding final value
  spec_RailP_pFlt : FromWorkspace  VariableName=testSig_RailP_pFlt  Interpolate=off  OutputAfterFinalValue=Holding final value
  spec_Rail_dvolDemSysMax : FromWorkspace  VariableName=testSig_Rail_dvolDemSysMax  Interpolate=off  OutputAfterFinalValue=Holding final value
  spec_Rail_dvolMeUnCtlUpLim : FromWorkspace  VariableName=testSig_Rail_dvolMeUnCtlUpLim  Interpolate=off  OutputAfterFinalValue=Holding final value
  spec_Rail_pDvt : FromWorkspace  VariableName=testSig_Rail_pDvt  Interpolate=off  OutputAfterFinalValue=Holding final value
  spec_Rail_pSetPoint : FromWorkspace  VariableName=testSig_Rail_pSetPoint  Interpolate=off  OutputAfterFinalValue=Holding final value
  spec_Rail_stCtlLoop : FromWorkspace  VariableName=testSig_Rail_stCtlLoop  Interpolate=off  OutputAfterFinalValue=Holding final value
  testSignals : Outport
  wires:
  BC/1 -> testSignals/1
  spec_Rail_pDvt/1 -> BC/1  "testSig_Rail_pDvt"
  spec_Epm_nEng/1 -> BC/2  "testSig_Epm_nEng"
  spec_MeUn_dvolSet/1 -> BC/3  "testSig_MeUn_dvolSet"
  spec_Rail_dvolMeUnCtlUpLim/1 -> BC/4  "testSig_Rail_dvolMeUnCtlUpLim"
  spec_Rail_stCtlLoop/1 -> BC/5  "testSig_Rail_stCtlLoop"
  spec_InjCtl_qSetUnBal/1 -> BC/6  "testSig_InjCtl_qSetUnBal"
  spec_FuelT_tFlSys/1 -> BC/7  "testSig_FuelT_tFlSys"
  spec_Rail_pSetPoint/1 -> BC/8  "testSig_Rail_pSetPoint"
  spec_Rail_dvolDemSysMax/1 -> BC/9  "testSig_Rail_dvolDemSysMax"
  spec_RailP_pFlt/1 -> BC/10  "testSig_RailP_pFlt"
  spec_MeUn_dvolSetAdapt/1 -> BC/11  "testSig_MeUn_dvolSetAdapt"
  spec_PthSet_stOvrRun/1 -> BC/12  "testSig_PthSet_stOvrRun"
  spec_APP_r/1 -> BC/13  "testSig_APP_r"
  spec_DSM_bRailMeUn0Rls/1 -> BC/14  "testSig_DSM_bRailMeUn0Rls"
  spec_DSM_bRailMeUn0Blk/1 -> BC/15  "testSig_DSM_bRailMeUn0Blk"
  spec_DSM_bRailMeUn2Rls/1 -> BC/16  "testSig_DSM_bRailMeUn2Rls"
  spec_DSM_bRailMeUn2Blk/1 -> BC/17  "testSig_DSM_bRailMeUn2Blk"
  spec_DSM_bRailMeUn22Rls/1 -> BC/18  "testSig_DSM_bRailMeUn22Rls"
  spec_DSM_bRailMeUn22Blk/1 -> BC/19  "testSig_DSM_bRailMeUn22Blk"
  spec_DSM_bRailMeUn3Rls/1 -> BC/20  "testSig_DSM_bRailMeUn3Rls"
  spec_DSM_bRailMeUn3Blk/1 -> BC/21  "testSig_DSM_bRailMeUn3Blk"
  spec_DSM_bRailMeUn4Rls/1 -> BC/22  "testSig_DSM_bRailMeUn4Rls"
  spec_DSM_bRailMeUn4Blk/1 -> BC/23  "testSig_DSM_bRailMeUn4Blk"
  spec_DSM_bRailMeUn42Rls/1 -> BC/24  "testSig_DSM_bRailMeUn42Rls"
  spec_DSM_bRailMeUn42Blk/1 -> BC/25  "testSig_DSM_bRailMeUn42Blk"
  spec_DSM_bRailMeUn7Rls/1 -> BC/26  "testSig_DSM_bRailMeUn7Rls"
  spec_DSM_bRailMeUn7Blk/1 -> BC/27  "testSig_DSM_bRailMeUn7Blk"
  spec_DSM_bRailMeUn8Rls/1 -> BC/28  "testSig_DSM_bRailMeUn8Rls"
  spec_DSM_bRailMeUn8Blk/1 -> BC/29  "testSig_DSM_bRailMeUn8Blk"
  spec_DSM_bRailMeUn10Rls/1 -> BC/30  "testSig_DSM_bRailMeUn10Rls"
  spec_DSM_bRailMeUn10Blk/1 -> BC/31  "testSig_DSM_bRailMeUn10Blk"
  spec_DFC_RailMeUn0_DSM/1 -> BC/32  "testSig_DFC_RailMeUn0_DSM"
  spec_DFC_RailMeUn2_DSM/1 -> BC/33  "testSig_DFC_RailMeUn2_DSM"
  spec_DFC_RailMeUn22_DSM/1 -> BC/34  "testSig_DFC_RailMeUn22_DSM"
  spec_DFC_RailMeUn3_DSM/1 -> BC/35  "testSig_DFC_RailMeUn3_DSM"
  spec_DFC_RailMeUn4_DSM/1 -> BC/36  "testSig_DFC_RailMeUn4_DSM"
  spec_DFC_RailMeUn42_DSM/1 -> BC/37  "testSig_DFC_RailMeUn42_DSM"
  spec_DFC_RailMeUn7_DSM/1 -> BC/38  "testSig_DFC_RailMeUn7_DSM"
  spec_DFC_RailMeUn8_DSM/1 -> BC/39  "testSig_DFC_RailMeUn8_DSM"
  spec_DFC_RailMeUn10_DSM/1 -> BC/40  "testSig_DFC_RailMeUn10_DSM"

== system TST_Rail_MonMeUn/simulationInput/testSignals_R004 ==
  BC : BusCreator  Inputs=40
  spec_APP_r : FromWorkspace  VariableName=testSig_APP_r  Interpolate=off  OutputAfterFinalValue=Holding final value
  spec_DFC_RailMeUn0_DSM : FromWorkspace  VariableName=testSig_DFC_RailMeUn0_DSM  Interpolate=off  OutputAfterFinalValue=Holding final value
  spec_DFC_RailMeUn10_DSM : FromWorkspace  VariableName=testSig_DFC_RailMeUn10_DSM  Interpolate=off  OutputAfterFinalValue=Holding final value
  spec_DFC_RailMeUn22_DSM : FromWorkspace  VariableName=testSig_DFC_RailMeUn22_DSM  Interpolate=off  OutputAfterFinalValue=Holding final value
  spec_DFC_RailMeUn2_DSM : FromWorkspace  VariableName=testSig_DFC_RailMeUn2_DSM  Interpolate=off  OutputAfterFinalValue=Holding final value
  spec_DFC_RailMeUn3_DSM : FromWorkspace  VariableName=testSig_DFC_RailMeUn3_DSM  Interpolate=off  OutputAfterFinalValue=Holding final value
  spec_DFC_RailMeUn42_DSM : FromWorkspace  VariableName=testSig_DFC_RailMeUn42_DSM  Interpolate=off  OutputAfterFinalValue=Holding final value
  spec_DFC_RailMeUn4_DSM : FromWorkspace  VariableName=testSig_DFC_RailMeUn4_DSM  Interpolate=off  OutputAfterFinalValue=Holding final value
  spec_DFC_RailMeUn7_DSM : FromWorkspace  VariableName=testSig_DFC_RailMeUn7_DSM  Interpolate=off  OutputAfterFinalValue=Holding final value
  spec_DFC_RailMeUn8_DSM : FromWorkspace  VariableName=testSig_DFC_RailMeUn8_DSM  Interpolate=off  OutputAfterFinalValue=Holding final value
  spec_DSM_bRailMeUn0Blk : FromWorkspace  VariableName=testSig_DSM_bRailMeUn0Blk  Interpolate=off  OutputAfterFinalValue=Holding final value
  spec_DSM_bRailMeUn0Rls : FromWorkspace  VariableName=testSig_DSM_bRailMeUn0Rls  Interpolate=off  OutputAfterFinalValue=Holding final value
  spec_DSM_bRailMeUn10Blk : FromWorkspace  VariableName=testSig_DSM_bRailMeUn10Blk  Interpolate=off  OutputAfterFinalValue=Holding final value
  spec_DSM_bRailMeUn10Rls : FromWorkspace  VariableName=testSig_DSM_bRailMeUn10Rls  Interpolate=off  OutputAfterFinalValue=Holding final value
  spec_DSM_bRailMeUn22Blk : FromWorkspace  VariableName=testSig_DSM_bRailMeUn22Blk  Interpolate=off  OutputAfterFinalValue=Holding final value
  spec_DSM_bRailMeUn22Rls : FromWorkspace  VariableName=testSig_DSM_bRailMeUn22Rls  Interpolate=off  OutputAfterFinalValue=Holding final value
  spec_DSM_bRailMeUn2Blk : FromWorkspace  VariableName=testSig_DSM_bRailMeUn2Blk  Interpolate=off  OutputAfterFinalValue=Holding final value
  spec_DSM_bRailMeUn2Rls : FromWorkspace  VariableName=testSig_DSM_bRailMeUn2Rls  Interpolate=off  OutputAfterFinalValue=Holding final value
  spec_DSM_bRailMeUn3Blk : FromWorkspace  VariableName=testSig_DSM_bRailMeUn3Blk  Interpolate=off  OutputAfterFinalValue=Holding final value
  spec_DSM_bRailMeUn3Rls : FromWorkspace  VariableName=testSig_DSM_bRailMeUn3Rls  Interpolate=off  OutputAfterFinalValue=Holding final value
  spec_DSM_bRailMeUn42Blk : FromWorkspace  VariableName=testSig_DSM_bRailMeUn42Blk  Interpolate=off  OutputAfterFinalValue=Holding final value
  spec_DSM_bRailMeUn42Rls : FromWorkspace  VariableName=testSig_DSM_bRailMeUn42Rls  Interpolate=off  OutputAfterFinalValue=Holding final value
  spec_DSM_bRailMeUn4Blk : FromWorkspace  VariableName=testSig_DSM_bRailMeUn4Blk  Interpolate=off  OutputAfterFinalValue=Holding final value
  spec_DSM_bRailMeUn4Rls : FromWorkspace  VariableName=testSig_DSM_bRailMeUn4Rls  Interpolate=off  OutputAfterFinalValue=Holding final value
  spec_DSM_bRailMeUn7Blk : FromWorkspace  VariableName=testSig_DSM_bRailMeUn7Blk  Interpolate=off  OutputAfterFinalValue=Holding final value
  spec_DSM_bRailMeUn7Rls : FromWorkspace  VariableName=testSig_DSM_bRailMeUn7Rls  Interpolate=off  OutputAfterFinalValue=Holding final value
  spec_DSM_bRailMeUn8Blk : FromWorkspace  VariableName=testSig_DSM_bRailMeUn8Blk  Interpolate=off  OutputAfterFinalValue=Holding final value
  spec_DSM_bRailMeUn8Rls : FromWorkspace  VariableName=testSig_DSM_bRailMeUn8Rls  Interpolate=off  OutputAfterFinalValue=Holding final value
  spec_Epm_nEng : FromWorkspace  VariableName=testSig_Epm_nEng  Interpolate=off  OutputAfterFinalValue=Holding final value
  spec_FuelT_tFlSys : FromWorkspace  VariableName=testSig_FuelT_tFlSys  Interpolate=off  OutputAfterFinalValue=Holding final value
  spec_InjCtl_qSetUnBal : FromWorkspace  VariableName=testSig_InjCtl_qSetUnBal  Interpolate=off  OutputAfterFinalValue=Holding final value
  spec_MeUn_dvolSet : FromWorkspace  VariableName=testSig_MeUn_dvolSet  Interpolate=off  OutputAfterFinalValue=Holding final value
  spec_MeUn_dvolSetAdapt : FromWorkspace  VariableName=testSig_MeUn_dvolSetAdapt  Interpolate=off  OutputAfterFinalValue=Holding final value
  spec_PthSet_stOvrRun : FromWorkspace  VariableName=testSig_PthSet_stOvrRun  Interpolate=off  OutputAfterFinalValue=Holding final value
  spec_RailP_pFlt : FromWorkspace  VariableName=testSig_RailP_pFlt  Interpolate=off  OutputAfterFinalValue=Holding final value
  spec_Rail_dvolDemSysMax : FromWorkspace  VariableName=testSig_Rail_dvolDemSysMax  Interpolate=off  OutputAfterFinalValue=Holding final value
  spec_Rail_dvolMeUnCtlUpLim : FromWorkspace  VariableName=testSig_Rail_dvolMeUnCtlUpLim  Interpolate=off  OutputAfterFinalValue=Holding final value
  spec_Rail_pDvt : FromWorkspace  VariableName=testSig_Rail_pDvt  Interpolate=off  OutputAfterFinalValue=Holding final value
  spec_Rail_pSetPoint : FromWorkspace  VariableName=testSig_Rail_pSetPoint  Interpolate=off  OutputAfterFinalValue=Holding final value
  spec_Rail_stCtlLoop : FromWorkspace  VariableName=testSig_Rail_stCtlLoop  Interpolate=off  OutputAfterFinalValue=Holding final value
  testSignals : Outport
  wires:
  BC/1 -> testSignals/1
  spec_Rail_pDvt/1 -> BC/1  "testSig_Rail_pDvt"
  spec_Epm_nEng/1 -> BC/2  "testSig_Epm_nEng"
  spec_MeUn_dvolSet/1 -> BC/3  "testSig_MeUn_dvolSet"
  spec_Rail_dvolMeUnCtlUpLim/1 -> BC/4  "testSig_Rail_dvolMeUnCtlUpLim"
  spec_Rail_stCtlLoop/1 -> BC/5  "testSig_Rail_stCtlLoop"
  spec_InjCtl_qSetUnBal/1 -> BC/6  "testSig_InjCtl_qSetUnBal"
  spec_FuelT_tFlSys/1 -> BC/7  "testSig_FuelT_tFlSys"
  spec_Rail_pSetPoint/1 -> BC/8  "testSig_Rail_pSetPoint"
  spec_Rail_dvolDemSysMax/1 -> BC/9  "testSig_Rail_dvolDemSysMax"
  spec_RailP_pFlt/1 -> BC/10  "testSig_RailP_pFlt"
  spec_MeUn_dvolSetAdapt/1 -> BC/11  "testSig_MeUn_dvolSetAdapt"
  spec_PthSet_stOvrRun/1 -> BC/12  "testSig_PthSet_stOvrRun"
  spec_APP_r/1 -> BC/13  "testSig_APP_r"
  spec_DSM_bRailMeUn0Rls/1 -> BC/14  "testSig_DSM_bRailMeUn0Rls"
  spec_DSM_bRailMeUn0Blk/1 -> BC/15  "testSig_DSM_bRailMeUn0Blk"
  spec_DSM_bRailMeUn2Rls/1 -> BC/16  "testSig_DSM_bRailMeUn2Rls"
  spec_DSM_bRailMeUn2Blk/1 -> BC/17  "testSig_DSM_bRailMeUn2Blk"
  spec_DSM_bRailMeUn22Rls/1 -> BC/18  "testSig_DSM_bRailMeUn22Rls"
  spec_DSM_bRailMeUn22Blk/1 -> BC/19  "testSig_DSM_bRailMeUn22Blk"
  spec_DSM_bRailMeUn3Rls/1 -> BC/20  "testSig_DSM_bRailMeUn3Rls"
  spec_DSM_bRailMeUn3Blk/1 -> BC/21  "testSig_DSM_bRailMeUn3Blk"
  spec_DSM_bRailMeUn4Rls/1 -> BC/22  "testSig_DSM_bRailMeUn4Rls"
  spec_DSM_bRailMeUn4Blk/1 -> BC/23  "testSig_DSM_bRailMeUn4Blk"
  spec_DSM_bRailMeUn42Rls/1 -> BC/24  "testSig_DSM_bRailMeUn42Rls"
  spec_DSM_bRailMeUn42Blk/1 -> BC/25  "testSig_DSM_bRailMeUn42Blk"
  spec_DSM_bRailMeUn7Rls/1 -> BC/26  "testSig_DSM_bRailMeUn7Rls"
  spec_DSM_bRailMeUn7Blk/1 -> BC/27  "testSig_DSM_bRailMeUn7Blk"
  spec_DSM_bRailMeUn8Rls/1 -> BC/28  "testSig_DSM_bRailMeUn8Rls"
  spec_DSM_bRailMeUn8Blk/1 -> BC/29  "testSig_DSM_bRailMeUn8Blk"
  spec_DSM_bRailMeUn10Rls/1 -> BC/30  "testSig_DSM_bRailMeUn10Rls"
  spec_DSM_bRailMeUn10Blk/1 -> BC/31  "testSig_DSM_bRailMeUn10Blk"
  spec_DFC_RailMeUn0_DSM/1 -> BC/32  "testSig_DFC_RailMeUn0_DSM"
  spec_DFC_RailMeUn2_DSM/1 -> BC/33  "testSig_DFC_RailMeUn2_DSM"
  spec_DFC_RailMeUn22_DSM/1 -> BC/34  "testSig_DFC_RailMeUn22_DSM"
  spec_DFC_RailMeUn3_DSM/1 -> BC/35  "testSig_DFC_RailMeUn3_DSM"
  spec_DFC_RailMeUn4_DSM/1 -> BC/36  "testSig_DFC_RailMeUn4_DSM"
  spec_DFC_RailMeUn42_DSM/1 -> BC/37  "testSig_DFC_RailMeUn42_DSM"
  spec_DFC_RailMeUn7_DSM/1 -> BC/38  "testSig_DFC_RailMeUn7_DSM"
  spec_DFC_RailMeUn8_DSM/1 -> BC/39  "testSig_DFC_RailMeUn8_DSM"
  spec_DFC_RailMeUn10_DSM/1 -> BC/40  "testSig_DFC_RailMeUn10_DSM"
